simulink model "datarecLAB3"  (R2020b)
settings: Solver=VariableStepAuto  StartTime=0.0  StopTime=20  RelTol=1e-3
values from neighbouring files (symbols this model uses):
  degs2rpm = 0.166666666667    [DIGIT1-BE20.mat]    (also in DIGIT1-BE4.mat; DIGIT1-TR4.mat; P2FFUOFF.mat; load_params_inertial_case.m)
  denF = [1 1.15847990004 0.419704605826]    [DIGIT1-BE20.mat]    (also in DIGIT1-BE4.mat = [1 -0.53010968182 0.221694090774]; DIGIT1-TR4.mat = [1 -0.53010968182 0.221694090774])
  filt =     [DIGIT1-BE20.mat]    (also in DIGIT1-BE4.mat; DIGIT1-TR4.mat; P2FFUOFF.mat)
  numF = [64.4546126467 0 -64.4546126467]    [DIGIT1-BE20.mat]    (also in DIGIT1-BE4.mat = [86.4480511192 0 -86.4480511192]; DIGIT1-TR4.mat = [86.4480511192 0 -86.4480511192])
  rpm2rads = 0.10471975512    [DIGIT1-BE20.mat]    (also in DIGIT1-BE4.mat; DIGIT1-TR4.mat; P2FFUOFF.mat; load_params_inertial_case.m)
  sens =     [DIGIT1-BE20.mat]    (also in DIGIT1-BE4.mat; DIGIT1-TR4.mat; P2FFUOFF.mat)
  Ts = 0.02    [DIGIT1-BE20.mat]    (also in DIGIT1-BE4.mat = 0.004; DIGIT1-TR4.mat = 0.004)
undefined symbols (not defined in the file or in its folder): National_Instruments, PCI
libraries: simulink x3, sldrtlib x3
settings Model: Creator=emanuelevitetta  LastModifiedBy=verrimarco
settings SolverCC: ZeroCrossAlgorithm=Adaptive
settings DebuggingCC: IgnoredZcDiagnostic=none  SFMachineParentedDataDiag=error

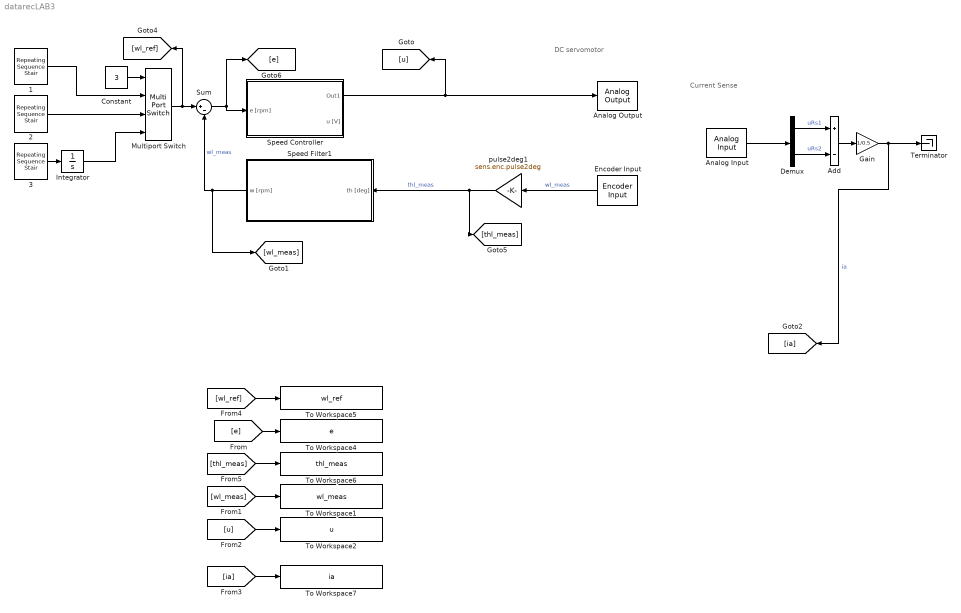
== system datarecLAB3 ==
  note: Current Sense
  note: DC servomotor
  1 : simulink/Sources/Repeating Sequence Stair  OutValues=[250 -250].'  tsamp=1.5  OutMin=[]  OutMax=[]  OutDataTypeStr=double  OutputDataTypeScalingMode=double  OutDataType=fixdt(0,8)  ConRadixGroup=Best Precision: Vector-wise  OutScaling=2^-12
  2 : simulink/Sources/Repeating Sequence Stair  OutValues=[0 50 100 150 200 250 300 350 400 450 ].'  tsamp=5  OutMin=[]  OutMax=[]  OutDataTypeStr=double  OutputDataTypeScalingMode=double  OutDataType=fixdt(0,8)  ConRadixGroup=Best Precision: Vector-wise  OutScaling=2^-12
  3 : simulink/Sources/Repeating Sequence Stair  OutValues=[450 -450].'  tsamp=1  OutMin=[]  OutMax=[]  OutDataTypeStr=double  OutputDataTypeScalingMode=double  OutDataType=fixdt(0,8)  ConRadixGroup=Best Precision: Vector-wise  OutScaling=2^-12
  Add : Sum  Inputs=+-
  Analog Input : sldrtlib/Analog Input  SampleTime=-1  MaxMissedTicks=10  ShowMissedTicks=off  YieldWhenWaiting=off  DrvName=National_Instruments/PCI-6221  DrvAddress=4294967295  DrvOptions=[0 0 0 2 0]  Channels=[1,2]  RangeMode=1  VoltRange=1  DataType=1
      settings: AttributesFormatString=National Instruments\nPCI-6221 [auto]
  Analog Output : sldrtlib/Analog Output  SampleTime=-1  MaxMissedTicks=10  ShowMissedTicks=off  YieldWhenWaiting=off  DrvName=National_Instruments/PCI-6221  DrvAddress=4294967295  DrvOptions=[0 0 0 2 0]  Channels=1  RangeMode=1  VoltRange=1  InitialValue=0  FinalValue=0
      settings: AttributesFormatString=National Instruments\nPCI-6221 [auto]
  Constant : Constant  Value=3
  Demux : Demux  Outputs=2
  Encoder Input : sldrtlib/Encoder Input  SampleTime=-1  MaxMissedTicks=10  ShowMissedTicks=off  YieldWhenWaiting=on  DrvName=National_Instruments/PCI-6221  DrvAddress=4294967295  DrvOptions=[0 0 0 2 0]  Channels=1  QuadMode=3  IndexPulse=1  InputFilter=Inf  DataType=1
      settings: AttributesFormatString=National Instruments\nPCI-6221 [auto]
  Gain : Gain  Gain=1/0.5
  Integrator : Integrator
  Multiport Switch : MultiPortSwitch
  Speed Controller : Subsystem
  Speed Filter1 : Subsystem
  Sum : Sum  Inputs=|+-
  Terminator : Terminator
  To Workspace1 : ToWorkspace  VariableName=wl_meas  SaveFormat=Structure With Time  SampleTime=-1
      settings: Save2DSignal=2-D array (concatenate along first dimension)
  To Workspace2 : ToWorkspace  VariableName=u  SaveFormat=Structure With Time  SampleTime=-1
      settings: Save2DSignal=2-D array (concatenate along first dimension)
  To Workspace4 : ToWorkspace  VariableName=e  SaveFormat=Structure With Time  SampleTime=-1
      settings: Save2DSignal=2-D array (concatenate along first dimension)
  To Workspace5 : ToWorkspace  VariableName=wl_ref  SaveFormat=Structure With Time  SampleTime=-1
      settings: Save2DSignal=2-D array (concatenate along first dimension)
  To Workspace6 : ToWorkspace  VariableName=thl_meas  SaveFormat=Structure With Time  SampleTime=-1
      settings: Save2DSignal=2-D array (concatenate along first dimension)
  To Workspace7 : ToWorkspace  VariableName=ia  SaveFormat=Structure With Time  SampleTime=-1
      settings: Save2DSignal=2-D array (concatenate along first dimension)
  pulse2deg1 : Gain  Gain=sens.enc.pulse2deg
  wires:
  Sum/1 -> [e], Speed Controller/1(e [rpm])
  Constant/1 -> Multiport Switch/1
  Multiport Switch/1 -> [wl_ref], Sum/1
  1/1 -> Multiport Switch/2
  2/1 -> Multiport Switch/3
  3/1 -> Integrator/1
  Integrator/1 -> Multiport Switch/4
  Demux/2 -> Add/2  "uRs2"
  Add/1 -> Gain/1
  Gain/1 -> [ia], Terminator/1  "ia"
  Analog Input/1 -> Demux/1
  Demux/1 -> Add/1  "uRs1"
  Speed Controller/1(Out1) -> [u], Analog Output/1
  Encoder Input/1 -> pulse2deg1/1  "wl_meas"
  [wl_ref] -> To Workspace5/1
  [u] -> To Workspace2/1
  [wl_meas] -> To Workspace1/1
  [thl_meas] -> To Workspace6/1
  [e] -> To Workspace4/1
  Speed Filter1/1(w [rpm]) -> [wl_meas], Sum/2  "wl_meas"
  pulse2deg1/1 -> [thl_meas], Speed Filter1/1(th [deg])  "thl_meas"
  [ia] -> To Workspace7/1

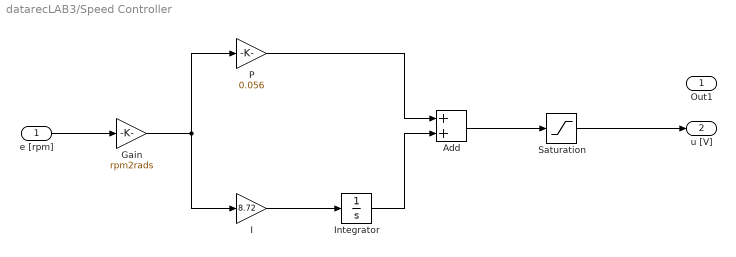
== system datarecLAB3/Speed Controller ==
  e [rpm] : Inport
  Add : Sum
  Gain : Gain  Gain=rpm2rads
  I : Gain  Gain=8.72
  Integrator : Integrator
  P : Gain  Gain=0.056
  Saturation : Saturate  UpperLimit=10  LowerLimit=-10
  Out1 : Outport
  u [V] : Outport  Port=2
  wires:
  e [rpm]/1 -> Gain/1
  I/1 -> Integrator/1
  P/1 -> Add/1
  Integrator/1 -> Add/2
  Add/1 -> Saturation/1
  Saturation/1 -> u [V]/1
  Gain/1 -> I/1, P/1

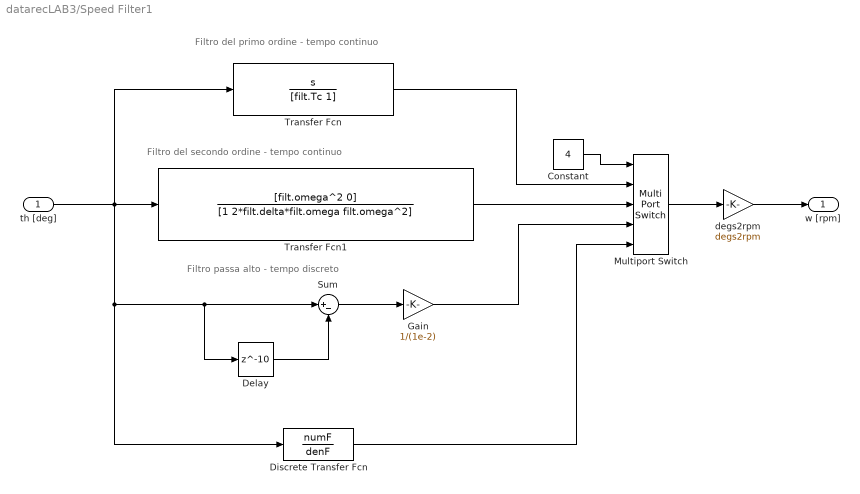
== system datarecLAB3/Speed Filter1 ==
  note: Filtro passa alto - tempo discreto
  note: Filtro del secondo ordine - tempo continuo
  note: Filtro del primo ordine - tempo continuo
  th [deg] : Inport
  Constant : Constant  Value=4
  Delay : Delay  DelayLength=10  InitialCondition=0
  Discrete Transfer Fcn : DiscreteTransferFcn  Numerator=numF  Denominator=denF  SampleTime=Ts
  Gain : Gain  Gain=1/(1e-2)
  Multiport Switch : MultiPortSwitch  Inputs=4
  Sum : Sum  Inputs=|+-
  Transfer Fcn : TransferFcn  Numerator=[1 0]  Denominator=[filt.Tc 1]
  Transfer Fcn1 : TransferFcn  Numerator=[filt.omega^2 0]  Denominator=[1 2*filt.delta*filt.omega filt.omega^2]
  degs2rpm : Gain  Gain=degs2rpm
  w [rpm] : Outport
  wires:
  degs2rpm/1 -> w [rpm]/1
  Transfer Fcn1/1 -> Multiport Switch/3
  Multiport Switch/1 -> degs2rpm/1
  Gain/1 -> Multiport Switch/4
  Delay/1 -> Sum/2
  Sum/1 -> Gain/1
  Constant/1 -> Multiport Switch/1
  Transfer Fcn/1 -> Multiport Switch/2
  th [deg]/1 -> Discrete Transfer Fcn/1, Delay/1, Sum/1, Transfer Fcn/1, Transfer Fcn1/1
  Discrete Transfer Fcn/1 -> Multiport Switch/5
